simulink model "SimulationDerRegelkreise"  (R2014b)
settings: Solver=ode45  StartTime=0.0  StopTime=30  RelTol=1e-3
libraries: vrlib x2
settings Model: Creator=Florian  LastModifiedBy=Florian

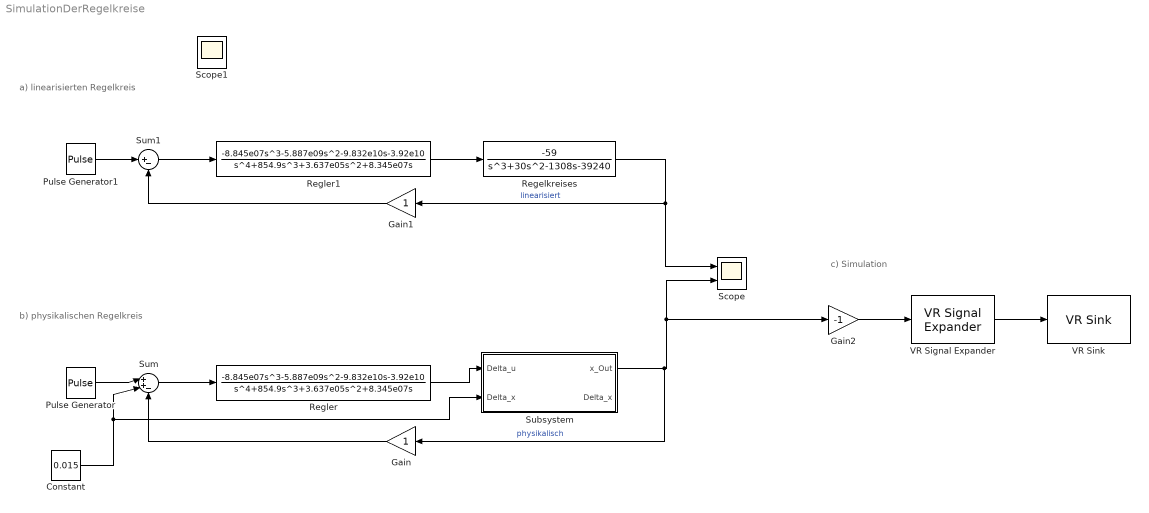
== system SimulationDerRegelkreise ==
  note: a) linearisierten Regelkreis
  note: b) physikalischen Regelkreis
  note: c) Simulation
  Constant : Constant  Value=0.015
  Gain : Gain
  Gain1 : Gain
  Gain2 : Gain  Gain=-1
  Pulse Generator : DiscretePulseGenerator  PulseType=Time based  Amplitude=0.001  Period=10  PulseWidth=50
  Pulse Generator1 : DiscretePulseGenerator  PulseType=Time based  Amplitude=0.001  Period=10  PulseWidth=50
  "Regelkreises " : TransferFcn  Numerator=[-59]  Denominator=[1 30 -1308 -39240]
  Regler : TransferFcn  Numerator=[-8.845e07 -5.887e09 -9.832e10 -3.92e10]  Denominator=[1 854.9 3.637e05 8.345e07 0]
  Regler1 : TransferFcn  Numerator=[-8.845e07 -5.887e09 -9.832e10 -3.92e10]  Denominator=[1 854.9 3.637e05 8.345e07 0]
  Scope : Scope  NumInputPorts=2
      settings: TimeRange=10  YMin=-0.0015~-1.5e+07  YMax=0.0025~-1.1e+07
  Subsystem : Subsystem  mask{x0=0.015, L=0.1, R=3}
  Sum : Sum  Inputs=|++-
  Sum1 : Sum  Inputs=|+-
  VR Signal Expander : vrlib/VR Signal Expander  outwidth=3  outidx=[2]
  VR Sink : vrlib/VR Sink  InstantiateOnLoad=on  SampleTime=0.1  ViewEnable=on  RemoteChange=off  RemoteView=off  FieldsWritten=Kugel.translation.3.1.1.double  WorldFileName=gegeben\Schwebekugel.WRL  AutoView=off  VideoDimensions=[]  AllowVariableSize=off  FigureProperties="{'Position', 'Name', 'Viewpoint', 'CameraBound', 'CameraDirection', 'CameraPosition', 'CameraUpVector', 'ZoomFactor', 'Antialiasing', 'Headlight', 'Lighting', 'NavPanel', 'Sound', 'StatusBar', 'Stereo3D', 'Stereo3DCameraOffset', 'Stereo3DHIT', 'ToolBar', 'Textures', 'Transparency', 'Triad', 'Wireframe', 'NavZones', 'NavMode', 'NavSpeed', 'CaptureFileFormat', 'CaptureFileName', 'Record2DCompressMethod', 'Record2DCompressQuality', 'Record2D', 'Record2DFileName', 'Record2DFPS'; [5.0000000000000000e+00   9.2000000000000000e+01   5.7600000000000000e+02   3.8000000000000000e+02], '', '_untitled_1', 'on', [0.0000000000000000e+00   0.0000000000000000e+00  -1.0000000000000000e+00], [0.0000000000000000e+00   0.0000000000000000e+00   0.0000000000000000e+00], [0.0000000000000000e+00   1.0000000000000000e+00   0.0000000000000000e+00], [1.7715610000000011e+00], 'on', 'on', 'on', 'halfbar', 'on', 'on', 'off', [1.0000000149011612e-01], [0.0000000000000000e+00], 'on', 'on', 'on', 'none', 'off', 'off', 'fly', 'normal', 'tif', '%f_anim_%n.tif', 'auto', [7.5000000000000000e+01], 'off', '%f_anim_%n.avi', 'auto'}"
  Scope1 : Scope
      settings: YMin=26  YMax=28.5
  wires:
  Pulse Generator/1 -> Sum/1
  Subsystem/1(x_Out) -> Gain/1, Gain2/1, Scope/2  "physikalisch"
  Sum/1 -> Regler/1
  Gain/1 -> Sum/3
  Regler/1 -> Subsystem/1(Delta_u)
  Pulse Generator1/1 -> Sum1/1
  "Regelkreises "/1 -> Scope/1, Gain1/1  "linearisiert"
  Gain1/1 -> Sum1/2
  Gain2/1 -> VR Signal Expander/1
  VR Signal Expander/1 -> VR Sink/1
  Sum1/1 -> Regler1/1
  Regler1/1 -> "Regelkreises "/1
  Constant/1 -> Subsystem/2("Delta_x "), Sum/2

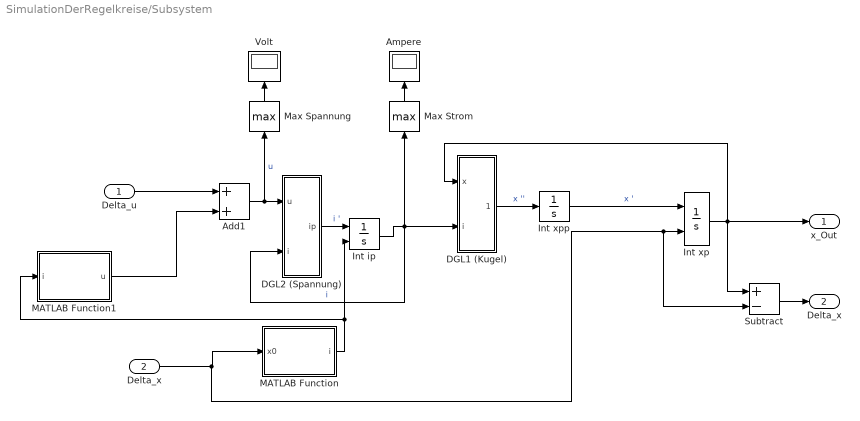
== system SimulationDerRegelkreise/Subsystem ==
  Delta_u : Inport
  "Delta_x " : Inport  Port=2
  Add1 : Sum
  Ampere : Display
  DGL1 (Kugel) : MATLAB Function  TreatAsAtomicUnit=on
  DGL2 (Spannung) : MATLAB Function  TreatAsAtomicUnit=on
  Int ip : Integrator  InitialConditionSource=external  InitialCondition=3.3221
  Int xp : Integrator  InitialConditionSource=external
  Int xpp : Integrator
  MATLAB Function : MATLAB Function  TreatAsAtomicUnit=on
  MATLAB Function1 : MATLAB Function  TreatAsAtomicUnit=on
  "Max Strom " : MinMax  Function=max
  Max Spannung : MinMax  Function=max
  Subtract : Sum  Inputs=+-
  Volt : Display
  x_Out : Outport
  Delta_x : Outport  Port=2
  wires:
  DGL2 (Spannung)/1(ip) -> Int ip/1  "i '"
  Int ip/1 -> DGL2 (Spannung)/2(i), "Max Strom "/1, DGL1 (Kugel)/2(i)  "i"
  DGL1 (Kugel)/1(xpp) -> Int xpp/1  "x ''"
  Int xpp/1 -> Int xp/1  "x '"
  Int xp/1 -> Subtract/1, x_Out/1, DGL1 (Kugel)/1(x)
  "Delta_x "/1 -> Subtract/2, Int xp/2, MATLAB Function/1(x0)
  Delta_u/1 -> Add1/1
  MATLAB Function1/1(u) -> Add1/2
  Add1/1 -> DGL2 (Spannung)/1(u), Max Spannung/1  "u"
  Subtract/1 -> Delta_x/1
  Max Spannung/1 -> Volt/1
  "Max Strom "/1 -> Ampere/1
  MATLAB Function/1(i) -> MATLAB Function1/1(i), Int ip/2

== matlab function SimulationDerRegelkreise/Subsystem/DGL1 (Kugel) ==
  data: x input; xpp output; i input
function xpp = fcn(x, i)

g = 9.81;    
m = 0.025;   
C = 5*10^-6; 

xpp = ((m*g)/m) - ((C*(i/x)^2)/m);

== matlab function SimulationDerRegelkreise/Subsystem/DGL2 (Spannung) ==
  data: u input; i input; ip output
function ip = fcn(u,i)

L = 0.1;
R = 3;   


ip = (u/L)  - ((R*i)/L);

== matlab function SimulationDerRegelkreise/Subsystem/MATLAB Function ==
  data: i output; x0 input
function i = fcn(x0)

m=0.025;
g=9.81;
c=5*10^-6;

i = sqrt((m*g)/c)*x0;

== matlab function SimulationDerRegelkreise/Subsystem/MATLAB Function1 ==
  data: u output; i input
function u = fcn(i)

R=3;


u = R*i;
